simulink model "forceFields"  (R2024b)
settings: Solver=FixedStepDiscrete  StartTime=0.0  StopTime=inf  FixedStep=0.001  RelTol=1e-3
libraries: PhanTorque_3Dof_Library_64Bits x2, simulink x1
settings Model: Creator=carlos.aldana  LastModifiedBy=elima
settings SolverCC: AlgebraicLoopSolver=TrustRegion
settings DataIOCC: LimitDataPoints=on  SaveFormat=Array  ReturnWorkspaceOutputs=off
settings OptimizationCC: BlockReduction=off  BooleanDataType=off  LifeSpan=inf
settings DebuggingCC: SaveWithParameterizedLinksMsg=none  UnderspecifiedInitializationDetection=Classic  MergeDetectMultiDrivingBlocksExec=none  SignalResolutionControl=TryResolveAllWithWarning  UnconnectedInputMsg=warning  UnconnectedOutputMsg=warning  UnconnectedLineMsg=warning  AllowSymbolicDim=off  SFUnexpectedBacktrackingDiag=warning  SFNoUnconditionalDefaultTransitionDiag=warning  SFExecutionAtInitializationDiag=none  ArithmeticOperatorsInVariantConditions=warning
settings HardwareCC: ProdBitPerPointer=32  ProdBitPerSizeT=32  ProdBitPerPtrDiffT=32  ProdLargestAtomicFloat=None  ProdIntDivRoundTo=Undefined  ProdEndianess=Unspecified  ProdWordSize=32  ProdHWDeviceType=32-bit Generic  TargetUnknown=on
settings ModelReferenceCC: EnableRefExpFcnMdlSchedulingChecks=on  PropagateSignalLabelsOutOfModel=off
settings SFSimCC: SimUseLocalCustomCode=off  CustomCodeUndefinedFunction=UseInterfaceOnly
settings RTWCC: RTWUseLocalCustomCode=off  GPUComputeCapability=3.5  DLArmComputeVersion=19.05
settings CodeAppCC: StateflowObjectComments=on
settings GRTTargetCC: TargetLangStandard=C89/C90 (ANSI)
settings ConfigComp: CovMetricSettings=dw  CovSaveCumulativeToWorkspaceVar=on  CovSaveSingleToWorkspaceVar=on  CovExternalEMLEnable=off  CovSFcnEnable=off

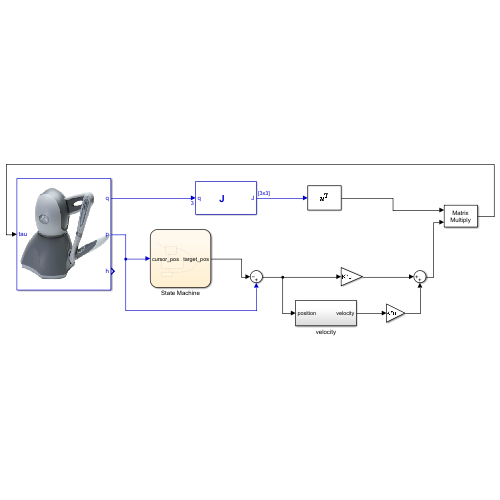
[thumbnail: Simulink's stored preview of the top-level diagram]
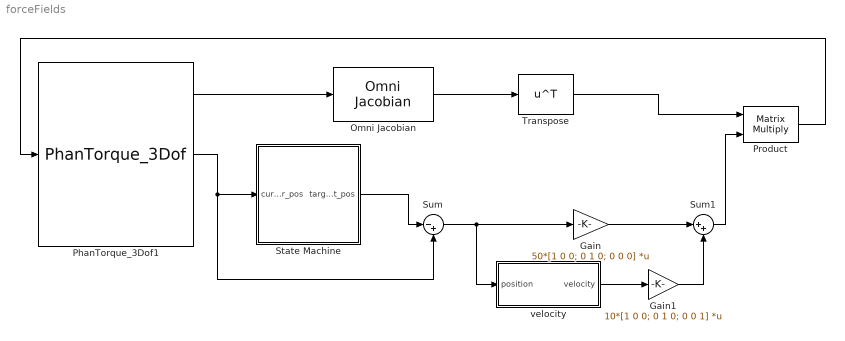
== system forceFields ==
  Gain : Gain  Gain=50*[1 0 0; 0 1 0; 0 0 0]  Multiplication=Matrix(K*u)
  Gain1 : Gain  Gain=10*[1 0 0; 0 1 0; 0 0 1]  Multiplication=Matrix(K*u)
  Omni Jacobian : PhanTorque_3Dof_Library_64Bits/Omni Jacobian  SystemSampleTime=-1  VariantActivationTime=update diagram  AllowFlexibleInterface=on  Latency=0  AutoFrameSizeCalculation=off
  PhanTorque_3Dof1 : PhanTorque_3Dof_Library_64Bits/PhanTorque_3Dof  Haptic_Name='Default Device'
  Product : Product  Multiplication=Matrix(*)
  State Machine : Stateflow chart  TreatAsAtomicUnit=on
  Sum : Sum  Inputs=|-+
  Sum1 : Sum  Inputs=|++
  Transpose : Math  Operator=transpose  SignedPower=on
  velocity : Subsystem
  wires:
  velocity/1(velocity) -> Gain1/1
  Gain/1 -> Sum1/1
  Gain1/1 -> Sum1/2
  PhanTorque_3Dof1/1 -> Omni Jacobian/1
  Omni Jacobian/1 -> Transpose/1
  Transpose/1 -> Product/1
  Sum1/1 -> Product/2
  Product/1 -> PhanTorque_3Dof1/1
  PhanTorque_3Dof1/2 -> State Machine/1(cursor_pos), Sum/2
  State Machine/1(target_pos) -> Sum/1
  Sum/1 -> velocity/1(position), Gain/1

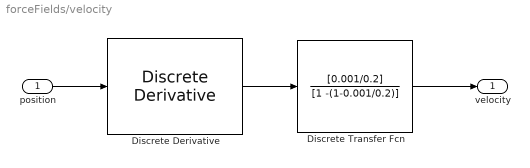
== system forceFields/velocity ==
  position : Inport
  Discrete Derivative : simulink/Discrete/Discrete Derivative  gainval=1.0  ICPrevScaledInput=0.0  OutMin=[]  OutMax=[]  OutDataType=fixdt(1, 16)  OutScaling=2^-10  DoSatur=off
  Discrete Transfer Fcn : DiscreteTransferFcn  Numerator=[0.001/0.2]  Denominator=[1 -(1-0.001/0.2)]
  velocity : Outport  VectorParamsAs1DForOutWhenUnconnected=off
  wires:
  position/1 -> Discrete Derivative/1
  Discrete Derivative/1 -> Discrete Transfer Fcn/1
  Discrete Transfer Fcn/1 -> velocity/1

== stateflow chart forceFields/State Machine ==
  settings: updateMethod=DISCRETE
  state Initializing
    entry:
    color = [0, 1, 1];
    target_pos = [0, 0, 0];
  state New_target
    entry:
    angle = counter * (pi/4);
    target_pos = [radius * cos(angle), radius * sin(angle), 0];
  state Finish
    entry:
    color = [0, 1, 0];
  (default) -> Initializing : {counter = 0}
  Finish -> Initializing : [after(1, sec) && counter < 7]{counter = counter + 1}
  Initializing -> New_target : [temporalCount(sec) >= 2 && double(norm(cursor_pos - target_pos)) < 1.0]
  New_target -> Finish : [double(norm(cursor_pos - target_pos)) < 1.0]
  data: target_pos output double size=[1 3]; cursor_pos input size=[1 3]; counter local; radius constant double =10; angle local double; color local double size=[1 3]
